simulink model "PTSD_single_channel_buffer"  (R2019b)
settings: Solver=VariableStepAuto  StartTime=0.0  StopTime=10  RelTol=1e-3
libraries: dspstat3 x2, simulink x2, dspswit3 x1
settings Model: Creator=sbuccelli  LastModifiedBy=sbuccelli

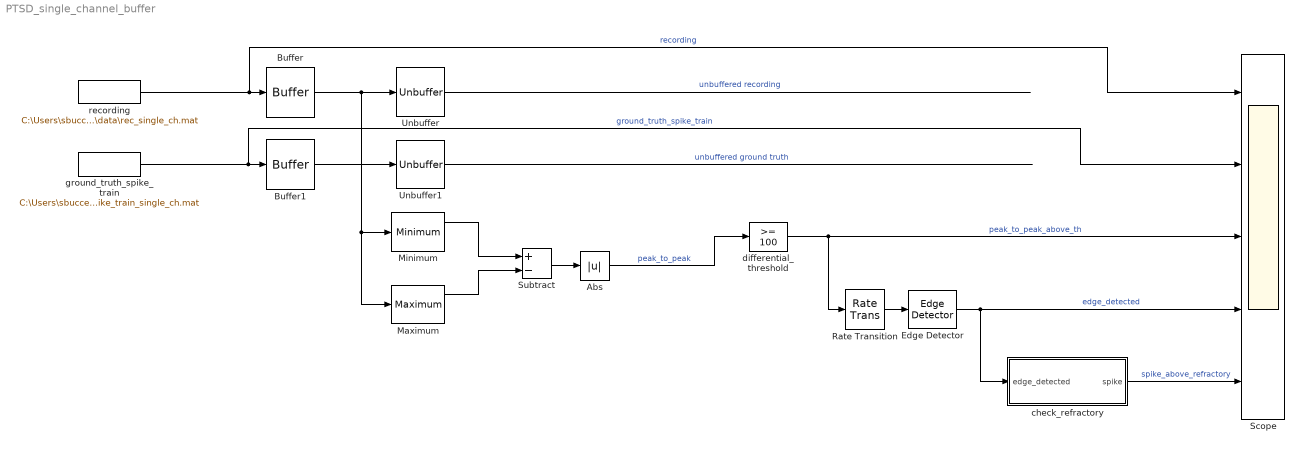
== system PTSD_single_channel_buffer ==
  Abs : Abs
  Buffer : Buffer  N=48  V=47  OutputFrames=off
  Buffer1 : Buffer  N=48  V=47  OutputFrames=off
  Edge Detector : dspswit3/Edge Detector  InputProcessing=Columns as channels (frame based)
      settings: SourceProductName=DSP System Toolbox  SourceProductBaseCode=DS
  Maximum : dspstat3/Maximum  operation=maximum  fcn=Value and Index  indexBase=One  operateOver=Each column  Dimension=1  InputProcessing=Columns as channels (frame based)  reset=None  roiEnable=off  roiType=Rectangles  roiPortion=Entire ROI  roiOutput=Individual statistics for each ROI  roiFlag=off  roundingMode=Floor  overflowMode=off  accumDataTypeStr=Inherit: Same as product output  accumLastDataTypeStr=Inherit: Same as product output
  Minimum : dspstat3/Minimum  operation=minimum  fcn=Value and Index  indexBase=One  operateOver=Each column  Dimension=1  InputProcessing=Columns as channels (frame based)  reset=None  roiEnable=off  roiType=Rectangles  roiPortion=Entire ROI  roiOutput=Individual statistics for each ROI  roiFlag=off  roundingMode=Floor  overflowMode=off
      settings: SourceProductName=DSP System Toolbox  SourceProductBaseCode=DS
  Rate Transition : RateTransition
  Scope : Scope  NumInputPorts=5
  Subtract : Sum  Inputs=+-
  Unbuffer : Unbuffer
  Unbuffer1 : Unbuffer
  check_refractory : Subsystem
  differential_threshold : simulink/Logic and Bit Operations/Compare To Constant  relop=>=  const=100  OutDataTypeStr=boolean
  ground_truth_spike_train : FromFile  FileName=C:\Users\sbuccelli\Documents\GitHub\closed-loop-neuroscience\data\spike_train_single_ch.mat  SampleTime=1/32e3
  recording : FromFile  FileName=C:\Users\sbuccelli\Documents\GitHub\closed-loop-neuroscience\data\rec_single_ch.mat  SampleTime=1/32e3
  wires:
  recording/1 -> Scope/1, Buffer/1  "recording"
  ground_truth_spike_train/1 -> Scope/2, Buffer1/1  "ground_truth_spike_train"
  differential_threshold/1 -> Rate Transition/1, Scope/3  "peak_to_peak_above_th"
  Edge Detector/1 -> check_refractory/1(edge_detected), Scope/4  "edge_detected"
  check_refractory/1(spike) -> Scope/5  "spike_above_refractory"
  Buffer/1 -> Maximum/1, Minimum/1, Unbuffer/1
  Buffer1/1 -> Unbuffer1/1
  Unbuffer/1 -> ?  "unbuffered recording"
  Unbuffer1/1 -> ?  "unbuffered ground truth"
  Minimum/1 -> Subtract/1
  Maximum/1 -> Subtract/2
  Subtract/1 -> Abs/1
  Abs/1 -> differential_threshold/1  "peak_to_peak"
  Rate Transition/1 -> Edge Detector/1

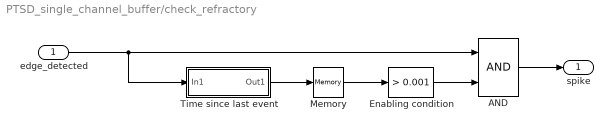
== system PTSD_single_channel_buffer/check_refractory ==
  edge_detected : Inport
  AND : Logic  IconShape=distinctive  AllPortsSameDT=off  OutDataTypeStr=boolean
  Enabling condition : simulink/Logic and Bit Operations/Compare To Constant  relop=>  const=0.001  OutDataTypeStr=boolean
  Memory : Memory  InheritSampleTime=on
  "Time since last event " : Subsystem
  spike : Outport
  wires:
  edge_detected/1 -> "Time since last event "/1(In1), AND/1
  Enabling condition/1 -> AND/2
  Memory/1 -> Enabling condition/1
  "Time since last event "/1(Out1) -> Memory/1
  AND/1 -> spike/1

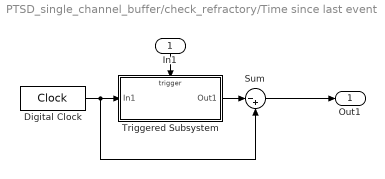
== system PTSD_single_channel_buffer/check_refractory/Time since last event  ==
  In1 : Inport
  Digital Clock : DigitalClock  SampleTime=1/32e3
  Sum : Sum  Inputs=|-+
  Triggered Subsystem : Subsystem  TreatAsAtomicUnit=on
  Out1 : Outport
  wires:
  Digital Clock/1 -> Sum/2, Triggered Subsystem/1(In1)
  Triggered Subsystem/1(Out1) -> Sum/1
  In1/1 -> Triggered Subsystem/Trigger
  Sum/1 -> Out1/1

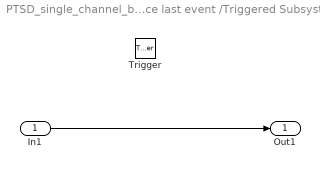
== system PTSD_single_channel_buffer/check_refractory/Time since last event /Triggered Subsystem ==
  In1 : Inport
  Trigger : TriggerPort  VariantControl=Variant
  Out1 : Outport
  wires:
  In1/1 -> Out1/1
